simulink model "Inv_Testing_v6"  (R2024b)
settings: Solver=FixedStepDiscrete  StartTime=0.0  StopTime=inf  FixedStep=0.002  RelTol=1e-3  EnableMultiTasking=on
PreLoadFcn:
  | % %--- PreStartFcn: initialize hold_flags.csv ---
  | % csvFile = '/Users/adamthompson/Desktop/Thesis/Motor Characterization V2/FPID_COMBINED_V1/Flags/hold_flags.csv';   % ← adjust to your real path
  | % fid = fopen(csvFile,'w');                      % open (or create) for overwrite
  | % if fid < 0
  | %     error('Cannot open flag file: %s', csvFile);
  | % end
  | % fprintf(fid, 'Index,SimTime_s\n');             % write header
  | % fclose(fid);
undefined symbols (not defined in the file or in its folder): outmax, outmin
libraries: arduinolib x8, fuzblock x2, arduinosensorlib x2, dspstat3 x2, mcbcontrolslib x1
settings Model: ExtModeTrigDuration=2  Creator=adamthompson  LastModifiedBy=adamthompson
settings SolverCC: AutoInsertRateTranBlk=on
settings OptimizationCC: BlockReduction=off  BooleanDataType=off  DefaultParameterBehavior=Inlined  EnhancedBackFolding=on  PassReuseOutputArgsAs=Individual arguments  ZeroExternalMemoryAtStartup=off  ZeroInternalMemoryAtStartup=off  MaxStackSize=64  OptimizeBlockOrder=speed  DifferentSizesBufferReuse=on  OptimizationCustomize=off  EfficientTunableParamExpr=on
settings DebuggingCC: SaveWithParameterizedLinksMsg=none  UnderspecifiedInitializationDetection=Classic  MergeDetectMultiDrivingBlocksExec=none  SignalResolutionControl=TryResolveAllWithWarning  ParameterTunabilityLossMsg=error
settings HardwareCC: ProdBitPerPointer=32  ProdBitPerSizeT=32  ProdBitPerPtrDiffT=32  ProdLargestAtomicInteger=Long  ProdLargestAtomicFloat=Double  ProdWordSize=32  ProdHWDeviceType=ARM Compatible->ARM Cortex
settings ModelReferenceCC: PropagateSignalLabelsOutOfModel=off
settings SFSimCC: MATLABDynamicMemAlloc=off
settings RTWCC: Description=Embedded Coder  SystemTargetFile=ert.tlc  HardwareBoard=Arduino Due  TemplateMakefile=ert_default_tmf  Toolchain=Arduino ARM  BuildConfiguration=Faster Runs
settings CodeAppCC: ForceParamTrailComments=on  IgnoreCustomStorageClasses=off  OperatorAnnotations=on  SimulinkDataObjDesc=on  SFDataObjDesc=on  InsertBlockDesc=on
settings ERTTargetCC: SupportContinuousTime=on  SupportVariableSizeSignals=on  ExtModeTransport=3  ExtModeStaticAlloc=on  ExtModeAutomaticAllocSize=off  ExtModeStaticAllocSize=24576  ExtModeMexFile=ext_xcp  ExtModeIntrfLevel=Level2 - Open

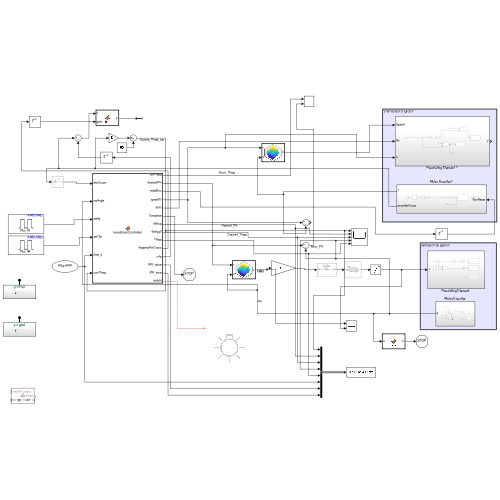
[thumbnail: Simulink's stored preview of the top-level diagram]
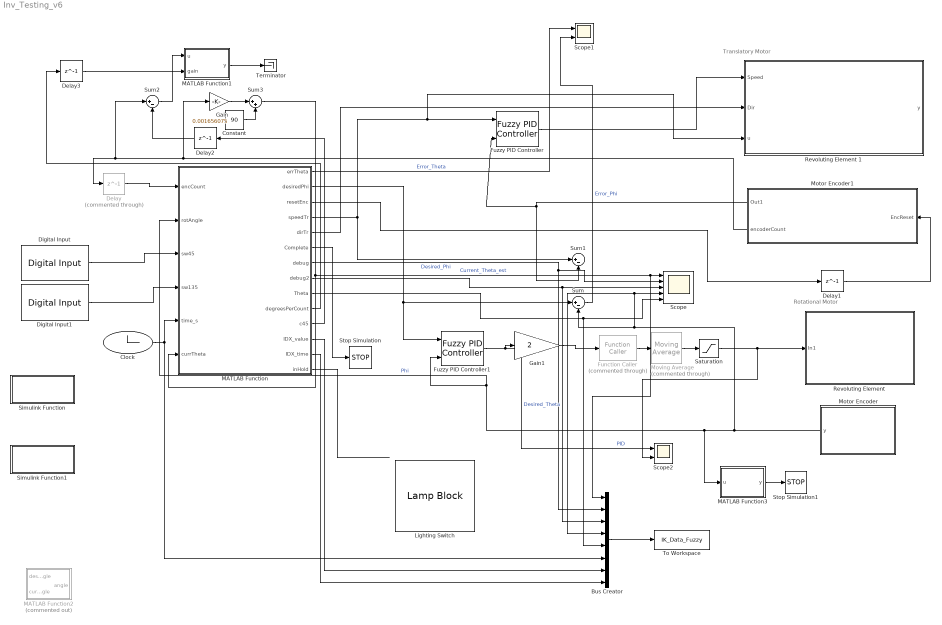
== system Inv_Testing_v6 ==
  note: Rotational Motor
  note: Translatory Motor
  Bus Creator : BusCreator  Inputs=8
  Clock : Clock
  Constant : Constant  Value=90
  Delay : Delay  Commented=through  DelayLength=1
  Delay1 : Delay  DelayLength=1
  Delay2 : Delay  DelayLength=1
  Delay3 : Delay  DelayLength=1
  Digital Input : arduinolib/Digital Input  pinNumber=51  mode=Input Pullup  Direction=input  SampleTime=-1  blockPlatform=arduino
  Digital Input1 : arduinolib/Digital Input  pinNumber=49  mode=Input Pullup  Direction=input  SampleTime=-1  blockPlatform=arduino
  Function Caller : FunctionCaller  Commented=through  FunctionPrototype=y = f(u)  InputArgumentSpecifications=<Enter example>  OutputArgumentSpecifications=<Enter example>
  Fuzzy PID Controller : fuzblock/Fuzzy PID Controller  TimeDomainType=Discrete-time  CE=10  CD=0.076335  C0=93.956  C1=9.3503  UseAccumulator=off  IntegratorMethod=Forward Euler  DerivativeSignal=Error (e)  UseFilter=off  N=100  DerivativeFilterMethod=Forward Euler  AddFFRefIn=off  E=off  SampleTime=-1  FIS=FIS  OutputSampleNumber=101  UseLookupTable=on  NumBreakpoints=20
  Fuzzy PID Controller1 : fuzblock/Fuzzy PID Controller  TimeDomainType=Discrete-time  CE=Ce  CD=Cd  C0=C0  C1=C1  UseAccumulator=off  IntegratorMethod=Forward Euler  DerivativeSignal=Error (e)  UseFilter=off  N=100  DerivativeFilterMethod=Forward Euler  AddFFRefIn=off  E=off  SampleTime=-1  FIS=fis_v4_1  OutputSampleNumber=101  UseLookupTable=on  NumBreakpoints=100
      link override FIS Variants/LookupTable/FIS: RemoveProtectionInput=on
  Gain : Gain  Gain=0.001656075
  Gain1 : Gain  Gain=2
  Lighting Switch : LampBlock  LabelPosition=Hide  Icon=LightingSwitch
  MATLAB Function : MATLAB Function  TreatAsAtomicUnit=on  SystemSampleTime=0.002
  MATLAB Function1 : MATLAB Function  TreatAsAtomicUnit=on
  MATLAB Function2 : MATLAB Function  Commented=on  TreatAsAtomicUnit=on
  MATLAB Function3 : MATLAB Function  TreatAsAtomicUnit=on
  Motor Encoder : Subsystem
  Motor Encoder1 : Subsystem
  Moving Average : dspstat3/Moving Average  Commented=through  Method=Exponential weighting  ForgettingFactorPort=off  SpecifyWindowLength=on  WindowLength=4  OverlapLength=3  AllowArbitraryInputLength=off  ForgettingFactor=0.99  SimulateUsing=Code generation
  "Revoluting Element " : Subsystem
  Revoluting Element 1 : Subsystem
  Saturation : Saturate  UpperLimit=200  LowerLimit=-200
  Scope : Scope  NumInputPorts=5
  Scope1 : Scope  NumInputPorts=2
  Scope2 : Scope  NumInputPorts=2
  Simulink Function : Subsystem  TreatAsAtomicUnit=on
  Simulink Function1 : Subsystem  TreatAsAtomicUnit=on
  Stop Simulation : Stop
  Stop Simulation1 : Stop
  Sum : Sum  Inputs=|+-
  Sum1 : Sum  Inputs=|+-
  Sum2 : Sum  Inputs=|+-
  Sum3 : Sum  Inputs=|++
  Terminator : Terminator
  To Workspace : ToWorkspace  VariableName=IK_Data_Fuzzy  SampleTime=-1
      settings: Save2DSignal=2-D array (concatenate along first dimension)
  wires:
  Saturation/1 -> Scope2/2, "Revoluting Element "/1(In1)
  Motor Encoder/1(y) -> MATLAB Function/2(rotAngle), Fuzzy PID Controller1/2, MATLAB Function3/1(u), Sum/2, Scope/4, Bus Creator/4  "Phi"
  Fuzzy PID Controller/1 -> Revoluting Element 1/1(Speed)
  Motor Encoder1/1(Out1) -> Sum1/2, Fuzzy PID Controller/2
  Motor Encoder1/2(encoderCount) -> Sum2/1, Delay/1, Gain/1
  Digital Input/1 -> MATLAB Function/3(sw45)
  Digital Input1/1 -> MATLAB Function/4(sw135)
  Clock/1 -> Bus Creator/6, MATLAB Function/5(time_s)
  MATLAB Function/5(dirTr) -> Revoluting Element 1/2(Dir)
  MATLAB Function/4(speedTr) -> Sum1/1, Fuzzy PID Controller/1, Revoluting Element 1/3(u)
  MATLAB Function/3(resetEnc) -> Delay1/1
  MATLAB Function/1(errTheta) -> Scope1/1  "Error_Theta"
  Delay/1 -> MATLAB Function/1(encCount)
  Delay1/1 -> Motor Encoder1/1(EncReset)
  MATLAB Function/6(Complete) -> Stop Simulation/1
  MATLAB Function/9(Theta) -> Scope/5, Bus Creator/5
  MATLAB Function/7(debug) -> Scope/2, Bus Creator/2  "Desired_Phi"
  MATLAB Function/8(debug2) -> Scope/3, Bus Creator/3  "Desired_Theta"
  Sum/1 -> Scope1/2  "Error_Phi"
  MATLAB Function/11(c45) -> Delay2/1
  MATLAB Function/10(degreesPerCount) -> Delay3/1
  Sum2/1 -> MATLAB Function1/1(u)
  Sum3/1 -> MATLAB Function/6(currTheta), Bus Creator/1, Scope/1  "Current_Theta_est"
  Constant/1 -> Sum3/2
  MATLAB Function1/1(y) -> Terminator/1
  Delay2/1 -> Sum2/2
  Delay3/1 -> MATLAB Function1/2(gain)
  Bus Creator/1 -> To Workspace/1
  MATLAB Function/12(IDX_value) -> Bus Creator/7
  MATLAB Function/13(IDX_time) -> Bus Creator/8
  MATLAB Function/14(inHold) -> ?
  Gain/1 -> Sum3/1
  Function Caller/1 -> Moving Average/1
  Moving Average/1 -> Saturation/1
  MATLAB Function3/1(y) -> Stop Simulation1/1
  Fuzzy PID Controller1/1 -> Scope2/1, Gain1/1  "PID"
  Gain1/1 -> Function Caller/1
  MATLAB Function/2(desiredPhi) -> Fuzzy PID Controller1/1, Sum/1

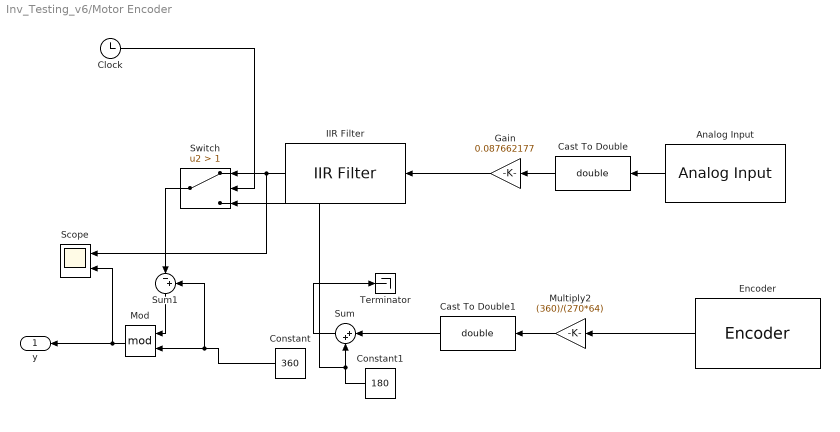
== system Inv_Testing_v6/Motor Encoder ==
  Analog Input : arduinolib/Analog Input  pinNumber=8  ReadResultsOnly=off  ConversionTriggerSource=Software  ExternalTriggerType=uint32( 0 )  OutputDataType=uint16  EnableConversionCompleteNotify=off  EnableOuputStatus=off  SampleTime=-1  blockPlatform=arduino
  Cast To Double : DataTypeConversion  OutDataTypeStr=double  SaturateOnIntegerOverflow=off  RndMeth=Floor
  Cast To Double1 : DataTypeConversion  OutDataTypeStr=double  SaturateOnIntegerOverflow=off  RndMeth=Floor
  Clock : Clock
  Constant : Constant  Value=360
  Constant1 : Constant  Value=180
  Encoder : arduinosensorlib/Encoder  InputA=7  InputB=6  Mode=No reset  SampleTime=-1
  Gain : Gain  Gain=0.087662177
  IIR Filter : mcbcontrolslib/IIR Filter  VariantControl=Low Pass Filter  VariantSelect=Low-pass  FilterConstantInputType=Specify via dialog  Filter_constant=0.01  advancedSettings=on  Ts=50e-6  cutOff_freq=32.1525
      settings: LibrarySourceBlock=mcbhdllib/Signal Management/IIR Filter
  Mod : Math  Operator=mod
  Multiply2 : Gain  Gain=(360)/(270*64)
  Scope : Scope  NumInputPorts=2
  Sum : Sum  Inputs=|++
  Sum1 : Sum  Inputs=|-+
  Switch : Switch  Criteria=u2 > Threshold  Threshold=1  SaturateOnIntegerOverflow=off  InputSameDT=off
  Terminator : Terminator
  y : Outport
  wires:
  Encoder/1 -> Multiply2/1
  Constant/1 -> Sum1/2, Mod/2
  Mod/1 -> Scope/2, y/1
  Multiply2/1 -> Cast To Double1/1
  Constant1/1 -> Sum/2, Switch/3
  Cast To Double1/1 -> Sum/1
  Sum/1 -> Terminator/1
  Cast To Double/1 -> Gain/1
  Analog Input/1 -> Cast To Double/1
  Gain/1 -> IIR Filter/1
  Clock/1 -> Switch/2
  IIR Filter/1 -> Scope/1, Switch/1
  Switch/1 -> Sum1/1
  Sum1/1 -> Mod/1

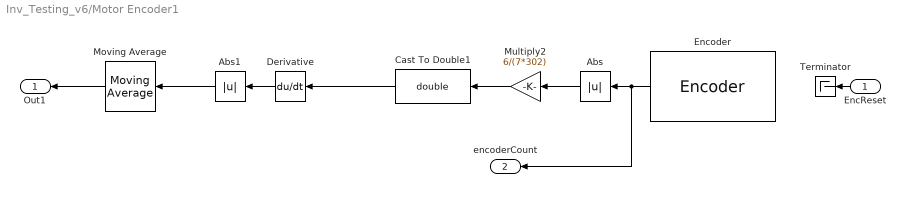
== system Inv_Testing_v6/Motor Encoder1 ==
  EncReset : Inport
  Abs : Abs  SaturateOnIntegerOverflow=off
  Abs1 : Abs  SaturateOnIntegerOverflow=off
  Cast To Double1 : DataTypeConversion  OutDataTypeStr=double  SaturateOnIntegerOverflow=off  RndMeth=Floor
  Derivative : Derivative
  Encoder : arduinosensorlib/Encoder  InputA=4  InputB=5  Mode=No reset  SampleTime=-1
  Moving Average : dspstat3/Moving Average  Method=Sliding window  ForgettingFactorPort=off  SpecifyWindowLength=on  WindowLength=4  OverlapLength=3  AllowArbitraryInputLength=off  ForgettingFactor=0.9  SimulateUsing=Code generation
  Multiply2 : Gain  Gain=6/(7*302)
  Terminator : Terminator
  Out1 : Outport
  encoderCount : Outport  Port=2
  wires:
  Encoder/1 -> encoderCount/1, Abs/1
  Cast To Double1/1 -> Derivative/1
  Abs/1 -> Multiply2/1
  Multiply2/1 -> Cast To Double1/1
  Derivative/1 -> Abs1/1
  Abs1/1 -> Moving Average/1
  Moving Average/1 -> Out1/1
  EncReset/1 -> Terminator/1

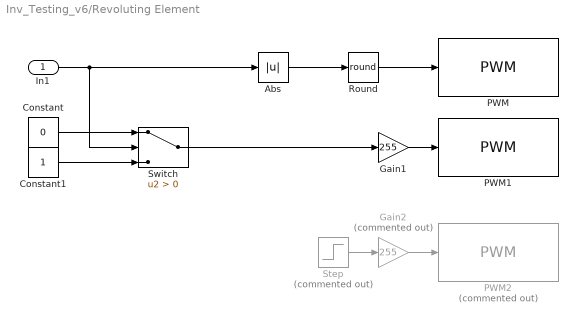
== system Inv_Testing_v6/Revoluting Element  ==
  In1 : Inport
  Abs : Abs  SaturateOnIntegerOverflow=off
  Constant : Constant  Value=0
  Constant1 : Constant
  Gain1 : Gain  Gain=255
  Gain2 : Gain  Commented=on  Gain=255
  PWM : arduinolib/PWM  pinNumber=11  frequencyType=Default  desiredFrequency=490.2  achievableFrequency=490.2
  PWM1 : arduinolib/PWM  pinNumber=13  frequencyType=Default  desiredFrequency=490.2  achievableFrequency=490.2
  PWM2 : arduinolib/PWM  Commented=on  pinNumber=8  frequencyType=Default  desiredFrequency=490.2  achievableFrequency=490.2
  Round : Rounding  Operator=round
  Step : Step  Commented=on  Time=8
  Switch : Switch  Criteria=u2 > Threshold  SaturateOnIntegerOverflow=off  InputSameDT=off
  wires:
  In1/1 -> Abs/1, Switch/2
  Gain1/1 -> PWM1/1
  Step/1 -> Gain2/1
  Gain2/1 -> PWM2/1
  Constant/1 -> Switch/1
  Constant1/1 -> Switch/3
  Switch/1 -> Gain1/1
  Abs/1 -> Round/1
  Round/1 -> PWM/1

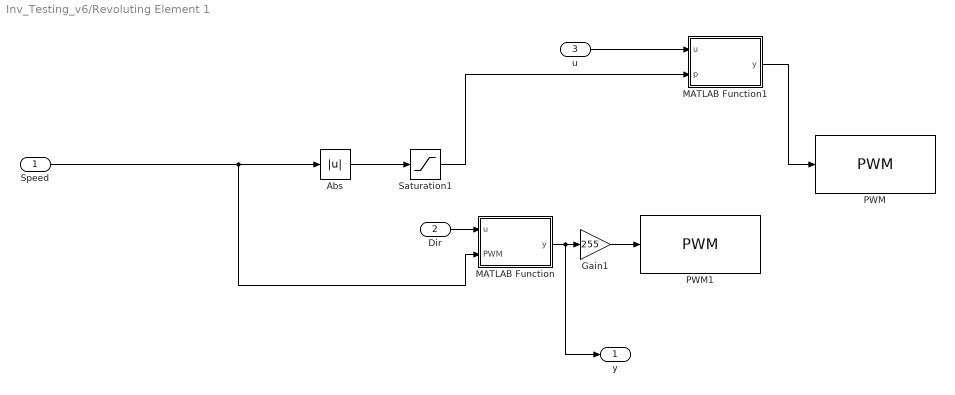
== system Inv_Testing_v6/Revoluting Element 1 ==
  Speed : Inport
  Dir : Inport  Port=2
  u : Inport  Port=3
  Abs : Abs  SaturateOnIntegerOverflow=off
  Gain1 : Gain  Gain=255
  MATLAB Function : MATLAB Function  TreatAsAtomicUnit=on
  MATLAB Function1 : MATLAB Function  TreatAsAtomicUnit=on
  PWM : arduinolib/PWM  pinNumber=3  frequencyType=Default  desiredFrequency=490.2  achievableFrequency=490.2
  PWM1 : arduinolib/PWM  pinNumber=12  frequencyType=Default  desiredFrequency=490.2  achievableFrequency=490.2
  Saturation1 : Saturate  UpperLimit=255  LowerLimit=0
  y : Outport
  wires:
  Gain1/1 -> PWM1/1
  Speed/1 -> MATLAB Function/2(PWM), Abs/1
  Abs/1 -> Saturation1/1
  Dir/1 -> MATLAB Function/1(u)
  MATLAB Function/1(y) -> y/1, Gain1/1
  u/1 -> MATLAB Function1/1(u)
  Saturation1/1 -> MATLAB Function1/2(p)
  MATLAB Function1/1(y) -> PWM/1

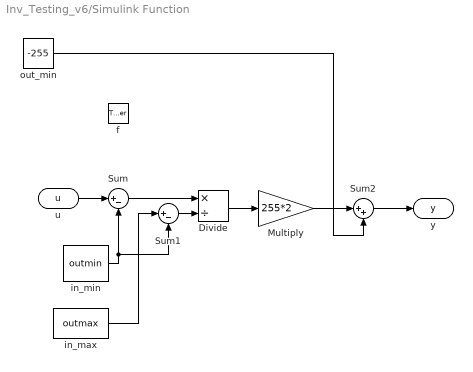
== system Inv_Testing_v6/Simulink Function ==
  f : TriggerPort  TriggerType=function-call  IsSimulinkFunction=on  FunctionName=f  FunctionVisibility=scoped  VariantControl=(inherit)
  Divide : Product  Inputs=*/
  Multiply : Gain  Gain=255*2
  Sum : Sum  Inputs=|+-
  Sum1 : Sum  Inputs=|+-
  Sum2 : Sum  Inputs=|++
  in_max : Constant  Value=outmax
  in_min : Constant  Value=outmin
  out_min : Constant  Value=-255
  u : ArgIn  DisableCoverage=on  ArgumentName=u
  y : ArgOut  DisableCoverage=on  ArgumentName=y
  wires:
  u/1 -> Sum/1
  in_min/1 -> Sum1/2, Sum/2
  Sum/1 -> Divide/1
  Sum1/1 -> Divide/2
  in_max/1 -> Sum1/1
  Divide/1 -> Multiply/1
  Multiply/1 -> Sum2/1
  Sum2/1 -> y/1
  out_min/1 -> Sum2/2

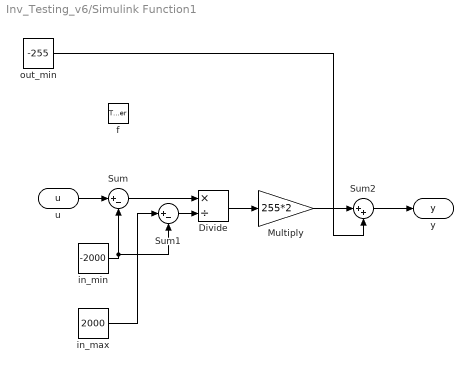
== system Inv_Testing_v6/Simulink Function1 ==
  f : TriggerPort  TriggerType=function-call  IsSimulinkFunction=on  FunctionName=g  FunctionVisibility=scoped  VariantControl=(inherit)
  Divide : Product  Inputs=*/
  Multiply : Gain  Gain=255*2
  Sum : Sum  Inputs=|+-
  Sum1 : Sum  Inputs=|+-
  Sum2 : Sum  Inputs=|++
  in_max : Constant  Value=2000
  in_min : Constant  Value=-2000
  out_min : Constant  Value=-255
  u : ArgIn  DisableCoverage=on  ArgumentName=u
  y : ArgOut  DisableCoverage=on  ArgumentName=y
  wires:
  u/1 -> Sum/1
  in_min/1 -> Sum1/2, Sum/2
  Sum/1 -> Divide/1
  Sum1/1 -> Divide/2
  in_max/1 -> Sum1/1
  Divide/1 -> Multiply/1
  Multiply/1 -> Sum2/1
  Sum2/1 -> y/1
  out_min/1 -> Sum2/2

== matlab function Inv_Testing_v6/Revoluting Element 1/MATLAB Function1 ==
  data: u input; y output; p input
function y = fcn(u, p)
if u == 0
    y = u;
else
    y = p;
end

== matlab function Inv_Testing_v6/MATLAB Function ==
  data: encCount input; errTheta output; rotAngle input; sw45 input; sw135 input; time_s input; desiredPhi output; resetEnc output; speedTr output; dirTr output; Complete output; debug output; debug2 output; Theta output; degreesPerCount output; c45 output; currTheta input; IDX_value output; IDX_time output; inHold output
function [errTheta, desiredPhi, resetEnc, speedTr, dirTr, Complete, debug, debug2, Theta, degreesPerCount, c45, IDX_value, IDX_time, inHold] = headScanController(encCount, rotAngle, sw45, sw135, time_s, currTheta)
% coder.extrinsic('set_param');
% headScanController  Five-state controller for translatory (θ) and rotational (φ) motors.
%
% Inputs:
%   encCount  – translatory motor encoder count
%   rotAngle  – current rotational motor angle φ (degrees)
%   sw45, sw135 – boolean inputs for 45° and 135° limit switches
%   time_s    – current time in seconds
%
% Outputs:
%   errTheta   – θ error (desiredθ – currentθ)
%   desiredPhi – desired φ
%   resetEnc   – true on the sample where encoder count should be zeroed
%   speedTr    – translatory motor speed (RPM)
%   dirTr      – translatory motor direction (1 = increasing count, 0 = decreasing)
%

%% PARAMETERS (tune or mask these)
persistent state degPerCount calCount45 calCount135 initTime holdStart idx phiTargets thetaTargets lastEnc lastTime valueList lastDesiredPhi thetaHoldStart lastDesiredTheta reachTimes ... 
    ku bu kd bd B velThresh pulseSamples lastS pulseCountdown lastX;
if isempty(state)
    state       = 1;           % 1=Calib,2=Init,3=Run,4=Hold,5=Done
    debug       = state;
    degPerCount = NaN;
    calCount135 = double(0);
    calCount45 = double(0); 
    idx         = 1;
    valueList = [-80 50
        -80 200
        80 200
        80 50
        -80 50
        -80 200
        80 200
        80 50];
   % valueList = [0 50
   %     0 75
   %     0 100 
   %     0 125
   %     0 150
   %     0 175
   %     0 200
   %     0 175
   %     0 150
   %     0 125
   %     0 100
   %     0 75
   %     0 50
   %     0 75
   %     0 100 
   %     0 125
   %     0 150
   %     0 175
   %     0 200
   %     0 175
   %     0 150
   %     0 125
   %     0 100
   %     0 75
   % %     0 50];
   % valueList = [-60 139.7
   %    -40 139.7
   %    -20 139.7
   %     0 139.7
   %     20 139.7
   %     40 139.7
   %     60 139.7
   %     80 139.7
   %     60 139.7
   %     40 139.7
   %     20 139.7
   %     0 139.7
   %     -20 139.7
   %     -40 139.7
   %     -60 139.7
   %     -80 139.7];
   
%    valueList = [-6.223012286	167.0642373
% -67.24044772	123.0712913
% -61.69999415	96.22438023
% -72.23192268	143.3872552
% 12.85236309	132.4313666
% 67.68066378	182.4138486
% 76.80060625	164.5579778
% 34.1895724	112.2947278
% 37.51407115	146.7406027
% -71.02956959	192.6766381
% -29.55771497	90.00696566
% -45.74437922	173.2836104
% -45.46746707	118.3758179
% 41.99283715	51.78027677
% 45.37136174	199.3113009
% -0.362311017	82.19487354
% -8.846660442	58.29168078
% 48.57564843	88.84331783
% 19.81897864	75.43023854
% -44.2980125	146.1256879
% -44.2980125	146.1256879
% 19.81897864	75.43023854
% 48.57564843	88.84331783
% -8.846660442	58.29168078
% -0.362311017	82.19487354
% 45.37136174	199.3113009
% 41.99283715	51.78027677
% -45.46746707	118.3758179
% -45.74437922	173.2836104
% -29.55771497	90.00696566
% -71.02956959	192.6766381
% 37.51407115	146.7406027
% 34.1895724	112.2947278
% 76.80060625	164.5579778
% 67.68066378	182.4138486
% 12.85236309	132.4313666
% -72.23192268	143.3872552
% -61.69999415	96.22438023
% -67.24044772	123.0712913
% -6.223012286	167.0642373];

    ku = 1.069487500454033;   bu = -1.120301764864740;   % <<< put your Inc-line slope/intercept
    kd = 0.926194701256995;  bd = -5.131311890884360;    % <<< put your Dec-line slope/intercept
    B  = 4.127904288140712;                      % <<< your estimated horizontal deadband
    velThresh    = 1.60e-04;            % small change threshold in x units
    pulseSamples = 1;              % 1 sample preload on reversals
    lastS = 0; pulseCountdown = 0; lastX = 0;
    lastEnc     = encCount;
    lastTime    = time_s;
    initTime    = 0;
    holdStart   = 0;
    Complete    = 0;
    inHold      = 0;
    desiredPhi = 180;
    lastDesiredPhi = desiredPhi;
    lastDesiredTheta = 90;
    thetaHoldStart = 0;

end

% Default outputs
resetEnc   = false;
speedTr    = 0;
dirTr      = 1;
desiredPhi = lastDesiredPhi;
desiredTheta = lastDesiredTheta; 
errTheta   = 0;
debug = 0;
debug2 = 0;
Complete    = 0;
inHold      = 0;
IDX_value = idx;
IDX_time = time_s;


% Compute current θ (only valid once degPerCount known)
if ~isnan(degPerCount)
    % currTheta = 45 + (encCount - calCount45)*degPerCount;
    Theta = currTheta;
    degreesPerCount = degPerCount;
    c45 = calCount45;
else
    % currTheta = int32(NaN);  
    Theta = currTheta;
    degreesPerCount = 0;
    c45 = 0;
end

switch state
  case 1  % CALIBRATION
    % Spin translatory motor until 135° switch
    speedTr = 10; dirTr = 1;
    desiredPhi = 180;
    if sw135
      speedTr = 0;
      calCount135 = double(encCount);
      % reverse direction
      dirTr = 0;
      state = 1.5;  % intermediate substate
    end

  case 1.5  % CALIBRATION reverse to 45°
    speedTr = 10; dirTr = 0;
    desiredPhi = 180;
    if sw45
      speedTr = 0;
      calCount45 = double(encCount);
      % compute degrees per count
      delta = abs(calCount135 - calCount45);
      degPerCount = 90 / delta;
      resetEnc   = true;               % reset Simulink count accumulator
      state      = 2;                  % go to INITIALIZATION
      initTime   = time_s;
    end

  case 2  % INITIALIZATION: move from 45° → 90°
    l = 177.8;   % Length to the base frame
    r = 139.7;   % Radius
    x_desired = -80.7930391251038; % Desired x-position
    y_desired = 139.7; % Desired y-position

    phi_rad = atan2(x_desired,l);
    theta_rad = atan2(l,(y_desired-r)*cos(phi_rad));
    desiredPhi = rad2deg(phi_rad)+180;
    
    % IDX_value = idx;
    % IDX_time = time_s;    
    lastDesiredPhi = desiredPhi; 
    desiredTheta = rad2deg(theta_rad);
    lastDesiredTheta = desiredTheta;
    debug = double(desiredPhi);
    debug2 = double(desiredTheta);
    % fprintf('Theta: %.4f radians\n', desiredTheta);
    % fprintf('Phi: %.4f radians\n', desiredPhi);
    % translatory
    errTheta = double(desiredTheta - currTheta);
    errPhi  = desiredPhi - rotAngle;
    speedTr  = 5;
    if desiredTheta < currTheta
        dirTr = 0;
    else
        dirTr = 1;
    end
    % stop translatory when close
    % --- inside your RUN case ---

    % check if θ has been within ±0.2 for at least 0.5 s
    if abs(errTheta) < 0.05
        speedTr = 0;
        errTheta = double(desiredTheta - currTheta);
        if thetaHoldStart == 0
            thetaHoldStart = time_s;        % start θ timer
        elseif time_s - thetaHoldStart >= 0.1
            % θ has been stable long enough → now check φ
            speedTr = 0;
            errPhi  = desiredPhi - rotAngle;
            if abs(errPhi) < 1.5
                errTheta = double(desiredTheta - currTheta);
                if holdStart == 0
                    holdStart = time_s;      % start φ timer
                elseif time_s - holdStart >= 10.0
                    state = 3;              % go to HOLD
                    holdStart = 0;          
                    thetaHoldStart = 0;     % reset for next cycle
                end
            else
                holdStart = 0;             % reset φ timer if φ out of range
            end
        end
    else
        % θ left the ±0.2 band → reset both timers
        thetaHoldStart = 0;
        holdStart      = 0;
        speedTr = 5; %* (errTheta/errPhi)
    end
    

  case 3  % RUN
    l = 177.8;   % Length to the base frame
    r = 139.7;   % Radius
    x_desired = valueList(idx,1); % Desired x-position
    y_desired = valueList(idx,2); % Desired y-position
    % ---- Backlash compensation on x_desired (manual constants) ----
    % di = x_desired - lastX;
    % if     di >  velThresh, s =  1;
    % elseif di < -velThresh, s = -1;
    % else,                   s =  lastS;
    % end
    % if s == 0, s = 1; end  % seed direction on first step
    % 
    % if s > 0
    %     base = (x_desired - bu) / max(ku, eps);
    % else
    %     base = (x_desired - bd) / max(kd, eps);
    % end
    % 
    % if (s ~= lastS) && (lastS ~= 0)
    %     pulseCountdown = pulseSamples;      % take-up on reversal
    % end
    % 
    % preload = 0;
    % if pulseCountdown > 0
    %     preload = s * B;
    %     pulseCountdown = pulseCountdown - 1;
    % end
    % 
    % x_cmd = base + preload;   % compensated command in x-units
    % lastS = s; 
    % lastX = x_desired;
    % ---------------------------------------------------------------
    phi_rad = atan2(x_desired,l);
    theta_rad = atan2(l,(y_desired-r)*cos(phi_rad));
    desiredPhi = rad2deg(phi_rad)+180;
    % if desiredPhi >180.4
    %     desiredPhi = desiredPhi - log(3*(desiredPhi-180));
    % elseif desiredPhi < 179.6
    %     desiredPhi = desiredPhi + log(3*(180-desiredPhi));
    % else
    %     desiredPhi = desiredPhi;
    % end
    
    % IDX_value = idx;
    % IDX_time = time_s;    
    lastDesiredPhi = desiredPhi; 
    desiredTheta = rad2deg(theta_rad);
    lastDesiredTheta = desiredTheta;
    debug = double(desiredPhi);
    debug2 = double(desiredTheta);
    % fprintf('Theta: %.4f radians\n', desiredTheta);
    % fprintf('Phi: %.4f radians\n', desiredPhi);
    % translatory
    errTheta = double(desiredTheta - currTheta);
    errPhi  = desiredPhi - rotAngle;
    speedTr  = 5;
    if desiredTheta < currTheta
        dirTr = 0;
    else
        dirTr = 1;
    end
    % stop translatory when close
    % --- inside your RUN case ---

    % check if θ has been within ±0.2 for at least 0.5 s
    if abs(errTheta) <= 0.05
        speedTr = 0;
        errTheta = double(desiredTheta - currTheta);
        if thetaHoldStart == 0
            thetaHoldStart = time_s;        % start θ timer
        elseif time_s - thetaHoldStart >= 0.5
            % θ has been stable long enough → now check φ
            speedTr = 0;
            errPhi  = desiredPhi - rotAngle;
            if abs(errPhi) < 1.5
                errTheta = double(desiredTheta - currTheta);
                if holdStart == 0
                    holdStart = time_s;      % start φ timer
                elseif time_s - holdStart >= 2
                    state = 4;              % go to HOLD
                    holdStart = 0;          
                    thetaHoldStart = 0;     % reset for next cycle
                end
            else
                holdStart = 0;             % reset φ timer if φ out of range
            end
        end
    else
        % θ left the ±0.2 band → reset both timers
        thetaHoldStart = 0;
        holdStart      = 0;
        speedTr = 5; %* (errTheta/errPhi)
    end

  case 4  % HOLD
    % hold both motors
    inHold      = 1;
    speedTr    = 0;
    desiredPhi = lastDesiredPhi;
    desiredTheta = lastDesiredTheta;
    debug = double(desiredPhi);
    debug2 = double(desiredTheta);
    IDX_value = idx;
    IDX_time = time_s;
    %desiredPhi = phiTargets(idx);
    if idx == 1
      reqHold = 2.1;    % first index: 1 second
    else
      reqHold = 2.0;    % later indices: 0.5 second
    end
    if holdStart == 0
      holdStart = time_s;
    elseif time_s - holdStart >= reqHold
      IDX_value = idx;
      IDX_time = holdStart;
      idx = idx + 1;
      holdStart = 0;
      if idx <= length(valueList)
        state = 3;  % next RUN
      else
        state = 5;  % DONE
      end
    
    end

  case 5  % DONE
    % return to home: θ→90°, φ→180°
    
    desiredPhi = 180;
    errTheta   = double(90 - currTheta);
    speedTr    = 5;
    dirTr      = double((errTheta > 0));
    if abs(errTheta) <= 0.01
        speedTr = 0;
        errTheta = double(desiredTheta - currTheta);
        if thetaHoldStart == 0
            thetaHoldStart = time_s;        % start θ timer
        elseif time_s - thetaHoldStart >= 0.5
            % θ has been stable long enough → now check φ
            speedTr = 0;
            errPhi  = desiredPhi - rotAngle;
            if abs(errPhi) < 3
                errTheta = double(desiredTheta - currTheta);
                if holdStart == 0
                    holdStart = time_s;      % start φ timer
                elseif time_s - holdStart >= 2
                    Complete = 1;              
                    holdStart = 0;          
                    thetaHoldStart = 0;     % reset for next cycle
                end
            else
                holdStart = 0;             % reset φ timer if φ out of range
            end
        end
    else
        % θ left the ±0.2 band → reset both timers
        thetaHoldStart = 0;
        holdStart      = 0;
        speedTr = 5; %* (errTheta/errPhi)
    end
end


% resetEnc only true on that one step after calibration
end

== matlab function Inv_Testing_v6/MATLAB Function1 ==
  data: u input; y output; gain input
function y = fcn(u, gain)

    y = u*gain;
    
end

== matlab function Inv_Testing_v6/MATLAB Function2 ==
  data: desired_angle input; current_angle input; angle output
function angle = step_plan_20deg(desired_angle, current_angle)
%#codegen
% Plans 20°-max steps whenever desired_angle changes.
% Output holds the current waypoint until the motor reaches it,
% then advances to the next. Final step snaps to desired if < 20°.
%
% Inputs : desired_angle [deg], current_angle [deg]   (0..360, no wrap)
% Output : angle [deg] (commanded setpoint)

% ---- Tunables ----
MAX_STEP = 10.0;    % deg
TOL_DEG  = 0.5;     % reach tolerance to advance to next step

% ---- Persistent state ----
persistent lastDesired steps stepCount idx dirSign initialized
if isempty(initialized)
    lastDesired = NaN;
    steps       = zeros(1,20);  % max needed: ceil(360/20)=18 (20 for safety)
    stepCount   = uint8(0);
    idx         = uint8(0);
    dirSign     = 0.0;
    initialized = true;
end

% Guard against bad inputs
if ~isfinite(desired_angle) || ~isfinite(current_angle)
    % Hold last target (or current if never initialized)
    if idx==0
        angle = current_angle;
    else
        angle = steps(double(idx));
    end
    return;
end

% ---- Re-plan if desired changed ----
if isnan(lastDesired) || abs(desired_angle - lastDesired) > 1e-9
    start = current_angle;                 % snapshot from where we are
    d     = desired_angle - start;         % signed delta (no wrap)
    ad    = abs(d);
    if ad < 1e-12
        % No movement needed
        stepCount = uint8(0);
        idx       = uint8(0);
        dirSign   = 0.0;
    else
        dirSign = sign(d);
        nFull   = floor(ad / MAX_STEP);    % number of full 20° steps
        remDeg  = ad - nFull*MAX_STEP;     % remainder (< 20°)

        % Build waypoints: nFull steps of 20°, plus final = desired if remainder
        k = 0;
        % full steps
        for i = 1:nFull
            k = k + 1;
            steps(k) = start + dirSign * (i*MAX_STEP);
        end
        % final remainder -> snap to desired (exact), if any
        if remDeg > 1e-9
            k = k + 1;
            steps(k) = desired_angle;
        end

        % Cap to buffer size (shouldn't be needed for 0..360)
        k = min(k, numel(steps));
        stepCount = uint8(k);
        idx       = uint8(1);
    end
    lastDesired = desired_angle;
end

% ---- Output & advance logic ----
if stepCount == 0
    % Nothing planned; command desired directly
    angle = desired_angle;
else
    tgt   = steps(double(idx));
    angle = tgt;

    % Consider reached if within tolerance or overshot in motion direction
    reached = (abs(current_angle - tgt) <= TOL_DEG) || ...
              (dirSign > 0 && current_angle >  tgt) || ...
              (dirSign < 0 && current_angle <  tgt);

    if reached && idx < stepCount
        idx = idx + 1;            % advance to next waypoint
        angle = steps(double(idx));
    end
end

% Keep command in [0,360)
angle = mod(angle, 360.0);

== matlab function Inv_Testing_v6/MATLAB Function3 ==
  data: u input; y output
function y = fcn(u)
    if (u>=270)||(u<=90)
        y = 1;
    else
        y = 0;
    end
end

== matlab function Inv_Testing_v6/Revoluting Element 1/MATLAB Function ==
  data: u input; y output; PWM input
function y = fcn(u, PWM)
    if (u == 1) && (PWM < 0)
        y = 0;
    elseif (u == 0) && (PWM < 0)
        y = 1;
    else
        y = u;
    end
    % y = u; %debug

end
